simulink model "lateralforce"  (R2015b)
settings: Solver=FixedStepAuto  StartTime=0.0  StopTime=1  FixedStep=0.001  RelTol=1e-3
libraries: simulink x3
settings Model: Creator=ADMIN  LastModifiedBy=ADMIN

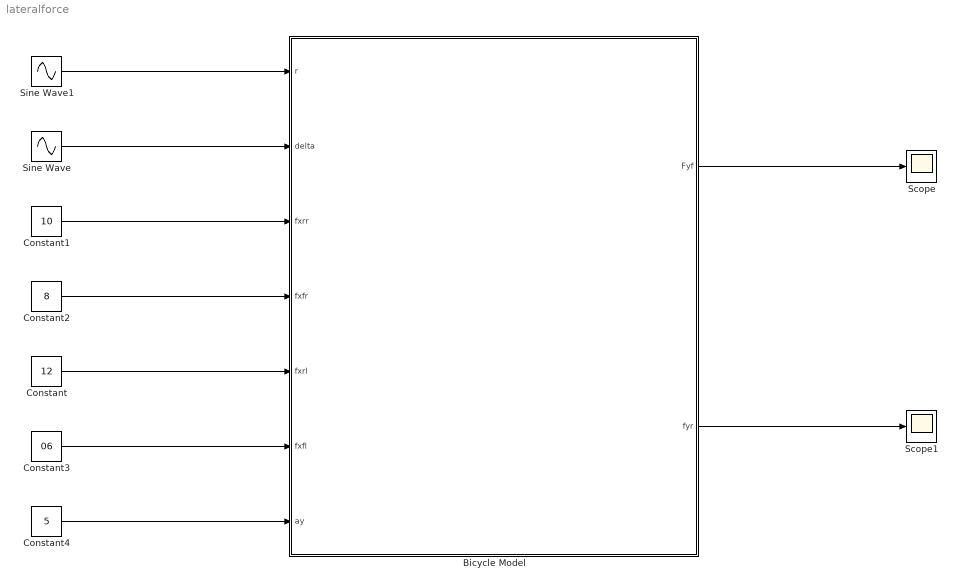
== system lateralforce ==
  Bicycle Model : Subsystem
  Constant : Constant  Value=12
  Constant1 : Constant  Value=10
  Constant2 : Constant  Value=8
  Constant3 : Constant  Value=06
  Constant4 : Constant  Value=5
  Scope : Scope
  Scope1 : Scope
  Sine Wave : Sin  Frequency=2
  Sine Wave1 : Sin  Frequency=4
  wires:
  Bicycle Model/1(Fyf) -> Scope/1
  Bicycle Model/2(fyr) -> Scope1/1
  Constant/1 -> Bicycle Model/5(fxrl)
  Sine Wave/1 -> Bicycle Model/2(delta)
  Constant3/1 -> Bicycle Model/6(fxfl)
  Constant2/1 -> Bicycle Model/4(fxfr)
  Constant1/1 -> Bicycle Model/3(fxrr)
  Constant4/1 -> Bicycle Model/7(ay)
  Sine Wave1/1 -> Bicycle Model/1(r)

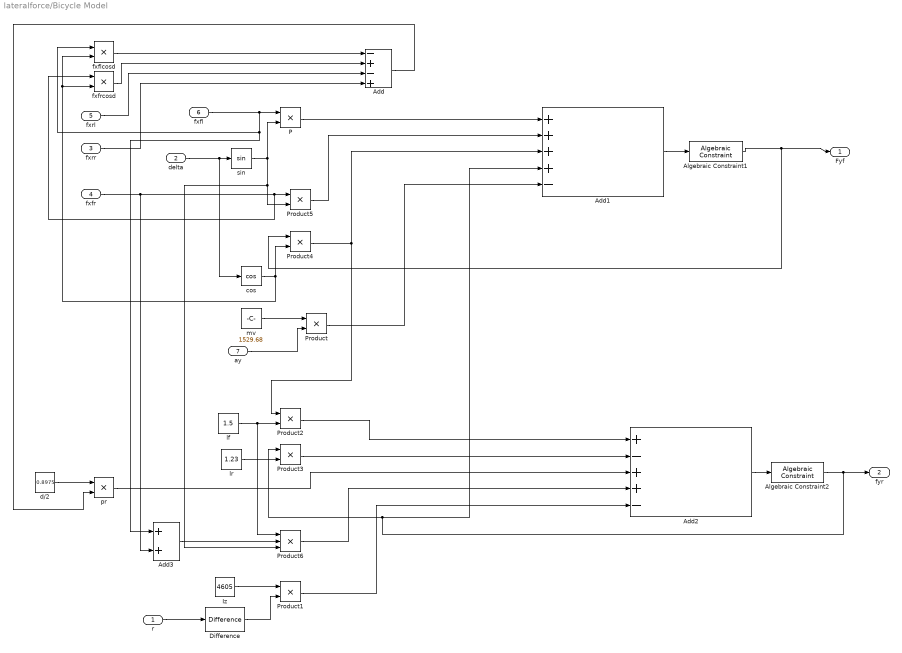
== system lateralforce/Bicycle Model ==
  r : Inport
  delta : Inport  Port=2
  fxrr : Inport  Port=3
  fxfr : Inport  Port=4
  fxrl : Inport  Port=5
  fxfl : Inport  Port=6
  ay : Inport  Port=7
  Add : Sum  Inputs=-+-+
  Add1 : Sum  Inputs=++++-
  Add2 : Sum  Inputs=+-++-
  Add3 : Sum
  Algebraic Constraint1 : simulink/Math Operations/Algebraic Constraint  z0=0
  Algebraic Constraint2 : simulink/Math Operations/Algebraic Constraint  z0=0
  Difference : simulink/Discrete/Difference  ICPrevInput=0.0  InputProcessing=Inherited  OutMin=[]  OutMax=[]  OutDataType=fixdt(1, 16)  OutScaling=2^-10  DoSatur=off
  Iz : Constant  Value=4605
  P : Product
  Product{,1..5} (6 alike) : Product
  Product6 : Product  Inputs=3
  cos : Trigonometry  Operator=cos
  d/2 : Constant  Value=0.8975
  fxflcosd : Product
  fxfrcosd : Product
  lf : Constant  Value=1.5
  lr : Constant  Value=1.23
  mv : Constant  Value=1529.68
  pr : Product
  sin : Trigonometry
  Fyf : Outport
  fyr : Outport  Port=2
  wires:
  fxfl/1 -> Add3/1, fxflcosd/1, P/1
  fxflcosd/1 -> Add/1
  Add3/1 -> Product6/2
  Add/1 -> pr/2
  Product6/1 -> Add2/4
  fxrr/1 -> Add/4
  fxrl/1 -> Add/3
  Product1/1 -> Add2/5
  fxfrcosd/1 -> Add/2
  r/1 -> Difference/1
  lr/1 -> Product3/2
  lf/1 -> Product6/1, Product2/2
  Product3/1 -> Add2/2
  Product2/1 -> Add2/1
  Iz/1 -> Product1/1
  Algebraic Constraint1/1 -> Product4/1, Fyf/1
  Algebraic Constraint2/1 -> Product3/1, Add1/4, fyr/1
  mv/1 -> Product/1
  ay/1 -> Product/2
  P/1 -> Add1/1
  delta/1 -> cos/1, sin/1
  Add1/1 -> Algebraic Constraint1/1
  Add2/1 -> Algebraic Constraint2/1
  fxfr/1 -> fxfrcosd/1, Product5/1, Add3/2
  sin/1 -> Product5/2, Product6/3, P/2
  Product5/1 -> Add1/2
  Product4/1 -> Product2/1, Add1/3
  cos/1 -> fxfrcosd/2, fxflcosd/2, Product4/2
  Product/1 -> Add1/5
  d/2/1 -> pr/1
  pr/1 -> Add2/3
  Difference/1 -> Product1/2
